simulink model "World_jessica_cs"  (R2019a)
settings: Solver=ode5  StartTime=0.0  StopTime=inf  FixedStep=1/60  RelTol=1e-3
PreLoadFcn:
  | mbxruntime.callbacks.PreLoadFcn(bdroot);
PostLoadFcn:
  | mbxruntime.callbacks.PostLoadFcn(bdroot);
InitFcn:
  | mbxruntime.callbacks.InitFcn(bdroot);
StartFcn:
  | mbxruntime.callbacks.StartFcn(bdroot);
StopFcn:
  | mbxruntime.callbacks.StopFcn(bdroot);
model workspace: external: MAT-File .\World_jessica_cs_hws.mat (data not in the file)
undefined symbols (not defined in the file or in its folder): DiscIntNeverNeededParam, InitImageOutputDir, mbxruntime, tabledata, World_jessica_cs_4acb408e0ac9f240, World_jessica_cs_800e508dbc53d9df, World_jessica_cs_Audi_A8_Sedan_1_Path_pathUniqueID, World_jessica_cs_bd1f9e0b3a3a0faa, World_jessica_cs_BMW_X5_SUV_1_Path_pathUniqueID, World_jessica_cs_BMW_X5_SUV_1_SpeedProfile_speedProfileUniqueID, World_jessica_cs_Boy_150_1_Path_pathUniqueID, World_jessica_cs_Boy_150_1_SpeedProfile_speedProfileUniqueID, World_jessica_cs_Citroen_C3_Hatchback_1_Path_pathUniqueID, World_jessica_cs_Male_CyclingCyclist_1_Path_pathUniqueID
libraries: adeye_lib x26, simulink_extras x24, simulink x2, PreScanUsefulBlocks x1
(part 5 of 7)

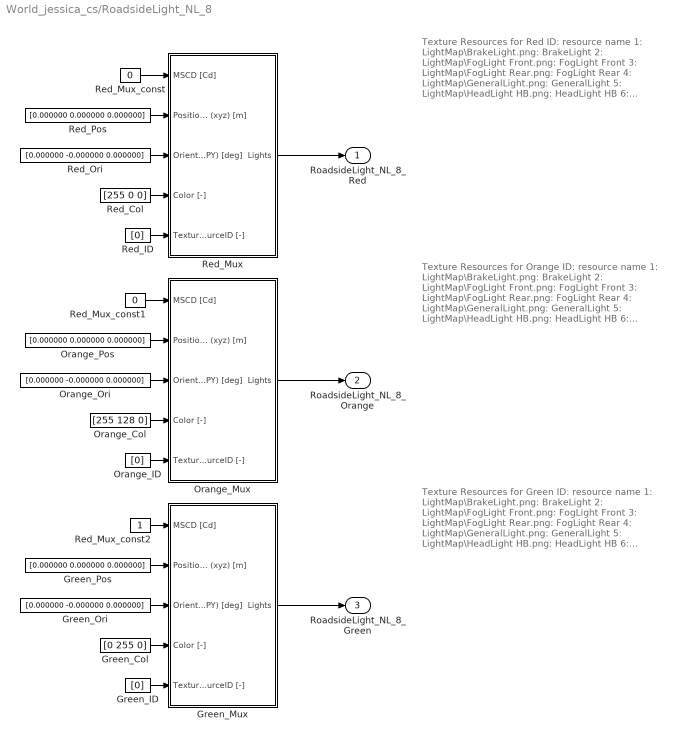
== system World_jessica_cs/RoadsideLight_NL_8 ==
  note: Texture Resources for Red
      |
      | ID: resource name
      | 1: LightMap\BrakeLight.png: BrakeLight
      | 2: LightMap\FogLight Front.png: FogLight Front
      | 3: LightMap\FogLight Rear.png: FogLight Rear
      | 4: LightMap\GeneralLight.png: GeneralLight
      | 5: LightMap\HeadLight HB.png: HeadLight HB
      | 6: LightMap\HeadLight LB.png: HeadLight LB
      | 7: LightMap\RearLight.png: RearLight
      | 8: LightMap\ReversingLight.png: ReversingLight
  note: Texture Resources for Orange
      |
      | ID: resource name
      | 1: LightMap\BrakeLight.png: BrakeLight
      | 2: LightMap\FogLight Front.png: FogLight Front
      | 3: LightMap\FogLight Rear.png: FogLight Rear
      | 4: LightMap\GeneralLight.png: GeneralLight
      | 5: LightMap\HeadLight HB.png: HeadLight HB
      | 6: LightMap\HeadLight LB.png: HeadLight LB
      | 7: LightMap\RearLight.png: RearLight
      | 8: LightMap\ReversingLight.png: ReversingLight
  note: Texture Resources for Green
      |
      | ID: resource name
      | 1: LightMap\BrakeLight.png: BrakeLight
      | 2: LightMap\FogLight Front.png: FogLight Front
      | 3: LightMap\FogLight Rear.png: FogLight Rear
      | 4: LightMap\GeneralLight.png: GeneralLight
      | 5: LightMap\HeadLight HB.png: HeadLight HB
      | 6: LightMap\HeadLight LB.png: HeadLight LB
      | 7: LightMap\RearLight.png: RearLight
      | 8: LightMap\ReversingLight.png: ReversingLight
  Green_Col : Constant  Tag=VisuLightConst  Value=[0 255 0]
  Green_ID : Constant  Tag=VisuLightConst  Value=[0]
  Green_Mux : Subsystem  Tag=mux/ActiveLight  mask(PreScan User Interface: VisuActiveLight){}
      mask help:
      | The VisuActiveLight block provides a way for detailed animation of Light Sources, such as the indicator, brake, fog and main lights of a vehicle, or a light post.
      |
      | For more information, please click Help.
      settings: DeleteFcn=PreScanBlockDeleteFcn;
      mask Help: eval('openHelp(209)')
  Green_Ori : Constant  Tag=VisuLightConst  Value=[0.000000 -0.000000 0.000000]
  Green_Pos : Constant  Tag=VisuLightConst  Value=[0.000000 0.000000 0.000000]
  Orange_Col : Constant  Tag=VisuLightConst  Value=[255 128 0]
  Orange_ID : Constant  Tag=VisuLightConst  Value=[0]
  Orange_Mux : Subsystem  Tag=mux/ActiveLight  mask(PreScan User Interface: VisuActiveLight){}
      mask help:
      | The VisuActiveLight block provides a way for detailed animation of Light Sources, such as the indicator, brake, fog and main lights of a vehicle, or a light post.
      |
      | For more information, please click Help.
      settings: DeleteFcn=PreScanBlockDeleteFcn;
      mask Help: eval('openHelp(209)')
  Orange_Ori : Constant  Tag=VisuLightConst  Value=[0.000000 -0.000000 0.000000]
  Orange_Pos : Constant  Tag=VisuLightConst  Value=[0.000000 0.000000 0.000000]
  Red_Col : Constant  Tag=VisuLightConst  Value=[255 0 0]
  Red_ID : Constant  Tag=VisuLightConst  Value=[0]
  Red_Mux : Subsystem  Tag=mux/ActiveLight  mask(PreScan User Interface: VisuActiveLight){}
      mask help:
      | The VisuActiveLight block provides a way for detailed animation of Light Sources, such as the indicator, brake, fog and main lights of a vehicle, or a light post.
      |
      | For more information, please click Help.
      settings: DeleteFcn=PreScanBlockDeleteFcn;
      mask Help: eval('openHelp(209)')
  Red_Mux_const : Constant  Tag=VisuLightConst  Value=0
  Red_Mux_const1 : Constant  Tag=VisuLightConst  Value=0
  Red_Mux_const2 : Constant  Tag=VisuLightConst
  Red_Ori : Constant  Tag=VisuLightConst  Value=[0.000000 -0.000000 0.000000]
  Red_Pos : Constant  Tag=VisuLightConst  Value=[0.000000 0.000000 0.000000]
  RoadsideLight_NL_8_Red : Outport  Tag=outport/Red  OutDataTypeStr=Bus: PRESCAN_VISULIGHTACTUATOR_DATA  SampleTime=1/60
  RoadsideLight_NL_8_Orange : Outport  Tag=outport/Orange  Port=2  OutDataTypeStr=Bus: PRESCAN_VISULIGHTACTUATOR_DATA  SampleTime=1/60
  RoadsideLight_NL_8_Green : Outport  Tag=outport/Green  Port=3  OutDataTypeStr=Bus: PRESCAN_VISULIGHTACTUATOR_DATA  SampleTime=1/60
  wires:
  Red_Mux_const/1 -> Red_Mux/1(MSCD [Cd])
  Red_Mux_const1/1 -> Orange_Mux/1(MSCD [Cd])
  Red_Mux_const2/1 -> Green_Mux/1(MSCD [Cd])
  Red_Mux/1(Lights) -> RoadsideLight_NL_8_Red/1
  Red_Pos/1 -> Red_Mux/2(Position (xyz) [m])
  Red_Ori/1 -> Red_Mux/3(Orientation (RPY) [deg])
  Red_Col/1 -> Red_Mux/4(Color [-])
  Red_ID/1 -> Red_Mux/5(TextureResourceID [-])
  Orange_Mux/1(Lights) -> RoadsideLight_NL_8_Orange/1
  Orange_Pos/1 -> Orange_Mux/2(Position (xyz) [m])
  Orange_Ori/1 -> Orange_Mux/3(Orientation (RPY) [deg])
  Orange_Col/1 -> Orange_Mux/4(Color [-])
  Orange_ID/1 -> Orange_Mux/5(TextureResourceID [-])
  Green_Mux/1(Lights) -> RoadsideLight_NL_8_Green/1
  Green_Pos/1 -> Green_Mux/2(Position (xyz) [m])
  Green_Ori/1 -> Green_Mux/3(Orientation (RPY) [deg])
  Green_Col/1 -> Green_Mux/4(Color [-])
  Green_ID/1 -> Green_Mux/5(TextureResourceID [-])

== system World_jessica_cs/RoadsideLight_NL_8_Green ==
  RoadsideLight_NL_8_Green : Inport  Tag=inport/Green  OutDataTypeStr=Bus: PRESCAN_VISULIGHTACTUATOR_DATA  SampleTime=1/60  BusOutputAsStruct=on
  Actuator : S-Function  FunctionName=sfun_VisuLightActuator  Parameters=mbxruntime.parameters.convert(UniqueID), mbxruntime.parameters.convert(LightName), mbxruntime.parameters.convert(PivotName), mbxruntime.parameters.convert(TextureResources), mbxruntime.parameters.convert(ColorsObjectName), mbxruntime.parameters.convert(MeshOnColor), mbxruntime.parameters.convert(MeshOffColor),tabledata, TimeStep  SFunctionDeploymentMode=off  EnableBusSupport=off  mask(PreScan Sink Block: VisuActiveLight){UniqueID=4882, LightName=RoadsideLight_NL_8.LightActuator_2_Green_ActiveLight, PivotName=RoadsideLight_NL_8.Green, TextureResources={ '1' 'LightMap\BrakeLight.png' '2' 'LightMap\FogLight Front.png' '3' 'LightMap\FogLight Rear.png' '4' 'LightMap\GeneralLight.png' '5' 'LightMap\HeadLight HB.png' '6' 'LightMap\HeadLight LB.png' '7' 'LightMap\RearLight.png' '8' 'LightMap\ReversingLight.png'}, ColorsObjectName=RoadsideLight_NL_8.Green, MeshOnColor=[0  100    0  255    0  100    0  255  102  102  102  255    0  510    0  255], MeshOffColor=[0  100    0  255    0  100    0  255  102  102  102  255    0    0    0  255], TimeStep=1/60}
      mask prompts: UniqueID "Parent Unique Identifier"; LightName "Light"; PivotName "Pivot"; TextureResources "Texture Resources"; ColorsObjectName "Light Fixture Color Object"; MeshOnColor "Light Fixture On Color"; MeshOffColor "Light Fixture Off Color"; TimeStep "Simulink time step"
      mask help:
      | The VisuActiveLight block provides a way for detailed animation of Light Sources, such as the indicator, brake, fog and main lights of a vehicle, or a light post.
      |
      | For more information, please click Help.
      mask init:
      | [tabledata] = mbxruntime.parameters.table(UniqueID,LightName,PivotName,TextureResources,ColorsObjectName,MeshOnColor,MeshOffColor);
      mask Help: eval('openHelp(209)')
      mask Display: image(imread('HeadLight.png'))
  wires:
  RoadsideLight_NL_8_Green/1 -> Actuator/1

== system World_jessica_cs/RoadsideLight_NL_8_Orange ==
  RoadsideLight_NL_8_Orange : Inport  Tag=inport/Orange  OutDataTypeStr=Bus: PRESCAN_VISULIGHTACTUATOR_DATA  SampleTime=1/60  BusOutputAsStruct=on
  Actuator : S-Function  FunctionName=sfun_VisuLightActuator  Parameters=mbxruntime.parameters.convert(UniqueID), mbxruntime.parameters.convert(LightName), mbxruntime.parameters.convert(PivotName), mbxruntime.parameters.convert(TextureResources), mbxruntime.parameters.convert(ColorsObjectName), mbxruntime.parameters.convert(MeshOnColor), mbxruntime.parameters.convert(MeshOffColor),tabledata, TimeStep  SFunctionDeploymentMode=off  EnableBusSupport=off  mask(PreScan Sink Block: VisuActiveLight){UniqueID=4882, LightName=RoadsideLight_NL_8.LightActuator_1_Orange_ActiveLight, PivotName=RoadsideLight_NL_8.Orange, TextureResources={ '1' 'LightMap\BrakeLight.png' '2' 'LightMap\FogLight Front.png' '3' 'LightMap\FogLight Rear.png' '4' 'LightMap\GeneralLight.png' '5' 'LightMap\HeadLight HB.png' '6' 'LightMap\HeadLight LB.png' '7' 'LightMap\RearLight.png' '8' 'LightMap\ReversingLight.png'}, ColorsObjectName=RoadsideLight_NL_8.Orange, MeshOnColor=[100   50    0  255  100   50    0  255  102  102  102  255  510  256    0  255], MeshOffColor=[100   50    0  255  100   50    0  255  102  102  102  255    0    0    0  255], TimeStep=1/60}
      mask prompts: UniqueID "Parent Unique Identifier"; LightName "Light"; PivotName "Pivot"; TextureResources "Texture Resources"; ColorsObjectName "Light Fixture Color Object"; MeshOnColor "Light Fixture On Color"; MeshOffColor "Light Fixture Off Color"; TimeStep "Simulink time step"
      mask help:
      | The VisuActiveLight block provides a way for detailed animation of Light Sources, such as the indicator, brake, fog and main lights of a vehicle, or a light post.
      |
      | For more information, please click Help.
      mask init:
      | [tabledata] = mbxruntime.parameters.table(UniqueID,LightName,PivotName,TextureResources,ColorsObjectName,MeshOnColor,MeshOffColor);
      mask Help: eval('openHelp(209)')
      mask Display: image(imread('HeadLight.png'))
  wires:
  RoadsideLight_NL_8_Orange/1 -> Actuator/1

== system World_jessica_cs/RoadsideLight_NL_8_Red ==
  RoadsideLight_NL_8_Red : Inport  Tag=inport/Red  OutDataTypeStr=Bus: PRESCAN_VISULIGHTACTUATOR_DATA  SampleTime=1/60  BusOutputAsStruct=on
  Actuator : S-Function  FunctionName=sfun_VisuLightActuator  Parameters=mbxruntime.parameters.convert(UniqueID), mbxruntime.parameters.convert(LightName), mbxruntime.parameters.convert(PivotName), mbxruntime.parameters.convert(TextureResources), mbxruntime.parameters.convert(ColorsObjectName), mbxruntime.parameters.convert(MeshOnColor), mbxruntime.parameters.convert(MeshOffColor),tabledata, TimeStep  SFunctionDeploymentMode=off  EnableBusSupport=off  mask(PreScan Sink Block: VisuActiveLight){UniqueID=4882, LightName=RoadsideLight_NL_8.LightActuator_0_Red_ActiveLight, PivotName=RoadsideLight_NL_8.Red, TextureResources={ '1' 'LightMap\BrakeLight.png' '2' 'LightMap\FogLight Front.png' '3' 'LightMap\FogLight Rear.png' '4' 'LightMap\GeneralLight.png' '5' 'LightMap\HeadLight HB.png' '6' 'LightMap\HeadLight LB.png' '7' 'LightMap\RearLight.png' '8' 'LightMap\ReversingLight.png'}, ColorsObjectName=RoadsideLight_NL_8.Red, MeshOnColor=[100    0    0  255  100    0    0  255  102  102  102  255  510    0    0  255], MeshOffColor=[100    0    0  255  100    0    0  255  102  102  102  255    0    0    0  255], TimeStep=1/60}
      mask prompts: UniqueID "Parent Unique Identifier"; LightName "Light"; PivotName "Pivot"; TextureResources "Texture Resources"; ColorsObjectName "Light Fixture Color Object"; MeshOnColor "Light Fixture On Color"; MeshOffColor "Light Fixture Off Color"; TimeStep "Simulink time step"
      mask help:
      | The VisuActiveLight block provides a way for detailed animation of Light Sources, such as the indicator, brake, fog and main lights of a vehicle, or a light post.
      |
      | For more information, please click Help.
      mask init:
      | [tabledata] = mbxruntime.parameters.table(UniqueID,LightName,PivotName,TextureResources,ColorsObjectName,MeshOnColor,MeshOffColor);
      mask Help: eval('openHelp(209)')
      mask Display: image(imread('HeadLight.png'))
  wires:
  RoadsideLight_NL_8_Red/1 -> Actuator/1

== system World_jessica_cs/SELF_Audi_A8_Sedan_1 ==
  Sensor : S-Function  FunctionName=sfun_SelfSensor  Parameters=UniqueID, TimeStep  SFunctionDeploymentMode=off  EnableBusSupport=off  mask(PreScan Source Block: SELF){UniqueID=4533, TimeStep=1/60}
      mask prompts: UniqueID "Auto-Assigned: Unique ID"; TimeStep "Auto-Assigned: Upload Period [s]"
      mask help:
      | The SELF port shows (state) information of the actor itself. The outputs are position in the experiment's axis system and the GPS coordinates, and the object's absolute velocity and compass heading.
      |
      | For more information, please click Help.
      mask Help: eval('openHelp(462)')
      mask Display: image(imread('GPS.png'))
  SELF_Audi_A8_Sedan_1 : Outport  Tag=outport/SelfPort  OutDataTypeStr=Bus: PRESCAN_SELFSENSORDATA  PortDimensions=1  SampleTime=1/60
  wires:
  Sensor/1 -> SELF_Audi_A8_Sedan_1/1

== system World_jessica_cs/SELF_BMW_X5_SUV_1 ==
  Sensor : S-Function  FunctionName=sfun_SelfSensor  Parameters=UniqueID, TimeStep  SFunctionDeploymentMode=off  EnableBusSupport=off  mask(PreScan Source Block: SELF){UniqueID=5671, TimeStep=1/60}
      mask prompts: UniqueID "Auto-Assigned: Unique ID"; TimeStep "Auto-Assigned: Upload Period [s]"
      mask help:
      | The SELF port shows (state) information of the actor itself. The outputs are position in the experiment's axis system and the GPS coordinates, and the object's absolute velocity and compass heading.
      |
      | For more information, please click Help.
      mask Help: eval('openHelp(462)')
      mask Display: image(imread('GPS.png'))
  SELF_BMW_X5_SUV_1 : Outport  Tag=outport/SelfPort  OutDataTypeStr=Bus: PRESCAN_SELFSENSORDATA  PortDimensions=1  SampleTime=1/60
  wires:
  Sensor/1 -> SELF_BMW_X5_SUV_1/1

== system World_jessica_cs/SELF_Boy_150_1 ==
  Sensor : S-Function  FunctionName=sfun_SelfSensor  Parameters=UniqueID, TimeStep  SFunctionDeploymentMode=off  EnableBusSupport=off  mask(PreScan Source Block: SELF){UniqueID=4541, TimeStep=1/60}
      mask prompts: UniqueID "Auto-Assigned: Unique ID"; TimeStep "Auto-Assigned: Upload Period [s]"
      mask help:
      | The SELF port shows (state) information of the actor itself. The outputs are position in the experiment's axis system and the GPS coordinates, and the object's absolute velocity and compass heading.
      |
      | For more information, please click Help.
      mask Help: eval('openHelp(462)')
      mask Display: image(imread('GPS.png'))
  SELF_Boy_150_1 : Outport  Tag=outport/SelfPort  OutDataTypeStr=Bus: PRESCAN_SELFSENSORDATA  PortDimensions=1  SampleTime=1/60
  wires:
  Sensor/1 -> SELF_Boy_150_1/1

== system World_jessica_cs/SELF_Citroen_C3_Hatchback_1 ==
  Sensor : S-Function  FunctionName=sfun_SelfSensor  Parameters=UniqueID, TimeStep  SFunctionDeploymentMode=off  EnableBusSupport=off  mask(PreScan Source Block: SELF){UniqueID=4537, TimeStep=1/60}
      mask prompts: UniqueID "Auto-Assigned: Unique ID"; TimeStep "Auto-Assigned: Upload Period [s]"
      mask help:
      | The SELF port shows (state) information of the actor itself. The outputs are position in the experiment's axis system and the GPS coordinates, and the object's absolute velocity and compass heading.
      |
      | For more information, please click Help.
      mask Help: eval('openHelp(462)')
      mask Display: image(imread('GPS.png'))
  SELF_Citroen_C3_Hatchback_1 : Outport  Tag=outport/SelfPort  OutDataTypeStr=Bus: PRESCAN_SELFSENSORDATA  PortDimensions=1  SampleTime=1/60
  wires:
  Sensor/1 -> SELF_Citroen_C3_Hatchback_1/1

== system World_jessica_cs/SELF_Male_CyclingCyclist_1 ==
  Sensor : S-Function  FunctionName=sfun_SelfSensor  Parameters=UniqueID, TimeStep  SFunctionDeploymentMode=off  EnableBusSupport=off  mask(PreScan Source Block: SELF){UniqueID=4545, TimeStep=1/60}
      mask prompts: UniqueID "Auto-Assigned: Unique ID"; TimeStep "Auto-Assigned: Upload Period [s]"
      mask help:
      | The SELF port shows (state) information of the actor itself. The outputs are position in the experiment's axis system and the GPS coordinates, and the object's absolute velocity and compass heading.
      |
      | For more information, please click Help.
      mask Help: eval('openHelp(462)')
      mask Display: image(imread('GPS.png'))
  SELF_Male_CyclingCyclist_1 : Outport  Tag=outport/SelfPort  OutDataTypeStr=Bus: PRESCAN_SELFSENSORDATA  PortDimensions=1  SampleTime=1/60
  wires:
  Sensor/1 -> SELF_Male_CyclingCyclist_1/1

== system World_jessica_cs/STATE_Audi_A8_Sedan_1_bus ==
  STATE_Audi_A8_Sedan_1_bus : Inport  Tag=inport/StatePort  OutDataTypeStr=Bus: PRESCAN_STATEACTUATORDATA  PortDimensions=1  SampleTime=1/60  BusOutputAsStruct=on
  Actuator : S-Function  FunctionName=sfun_StateActuator  Parameters=UniqueID, TimeStep  SFunctionDeploymentMode=off  EnableBusSupport=off  mask(PreScan Sink Block: State){UniqueID=4533, TimeStep=1/60}
      mask prompts: UniqueID "Auto-Assigned: Unique ID"; TimeStep "Auto-Assigned: Upload Period [s]"
      mask help:
      | The Actor State contains a vector signal of size (9x1), containing the following signals:
      |
      | -  Position    	(x,y,z)             	[m]
      | -  Velocity    	(vx,vy,vz)         	[m/s]
      | -  Angles       	(Roll, Pitch, Yaw)	[rad]
      |
      | The Actor state is defined in the global axis system.
      | The state is superponed on the Initial position defined in the GUI.
      |
      | For more information, please click Help.
      mask Help: eval('openHelp(222)')
      mask Display: image(imread('State.png'))
  wires:
  STATE_Audi_A8_Sedan_1_bus/1 -> Actuator/1

== system World_jessica_cs/STATE_BMW_X5_SUV_1_bus ==
  STATE_BMW_X5_SUV_1_bus : Inport  Tag=inport/StatePort  OutDataTypeStr=Bus: PRESCAN_STATEACTUATORDATA  PortDimensions=1  SampleTime=1/60  BusOutputAsStruct=on
  Actuator : S-Function  FunctionName=sfun_StateActuator  Parameters=UniqueID, TimeStep  SFunctionDeploymentMode=off  EnableBusSupport=off  mask(PreScan Sink Block: State){UniqueID=5671, TimeStep=1/60}
      mask prompts: UniqueID "Auto-Assigned: Unique ID"; TimeStep "Auto-Assigned: Upload Period [s]"
      mask help:
      | The Actor State contains a vector signal of size (9x1), containing the following signals:
      |
      | -  Position    	(x,y,z)             	[m]
      | -  Velocity    	(vx,vy,vz)         	[m/s]
      | -  Angles       	(Roll, Pitch, Yaw)	[rad]
      |
      | The Actor state is defined in the global axis system.
      | The state is superponed on the Initial position defined in the GUI.
      |
      | For more information, please click Help.
      mask Help: eval('openHelp(222)')
      mask Display: image(imread('State.png'))
  wires:
  STATE_BMW_X5_SUV_1_bus/1 -> Actuator/1

== system World_jessica_cs/STATE_Boy_150_1_bus ==
  STATE_Boy_150_1_bus : Inport  Tag=inport/StatePort  OutDataTypeStr=Bus: PRESCAN_STATEACTUATORDATA  PortDimensions=1  SampleTime=1/60  BusOutputAsStruct=on
  Actuator : S-Function  FunctionName=sfun_StateActuator  Parameters=UniqueID, TimeStep  SFunctionDeploymentMode=off  EnableBusSupport=off  mask(PreScan Sink Block: State){UniqueID=4541, TimeStep=1/60}
      mask prompts: UniqueID "Auto-Assigned: Unique ID"; TimeStep "Auto-Assigned: Upload Period [s]"
      mask help:
      | The Actor State contains a vector signal of size (9x1), containing the following signals:
      |
      | -  Position    	(x,y,z)             	[m]
      | -  Velocity    	(vx,vy,vz)         	[m/s]
      | -  Angles       	(Roll, Pitch, Yaw)	[rad]
      |
      | The Actor state is defined in the global axis system.
      | The state is superponed on the Initial position defined in the GUI.
      |
      | For more information, please click Help.
      mask Help: eval('openHelp(222)')
      mask Display: image(imread('State.png'))
  wires:
  STATE_Boy_150_1_bus/1 -> Actuator/1

== system World_jessica_cs/STATE_Citroen_C3_Hatchback_1_bus ==
  STATE_Citroen_C3_Hatchback_1_bus : Inport  Tag=inport/StatePort  OutDataTypeStr=Bus: PRESCAN_STATEACTUATORDATA  PortDimensions=1  SampleTime=1/60  BusOutputAsStruct=on
  Actuator : S-Function  FunctionName=sfun_StateActuator  Parameters=UniqueID, TimeStep  SFunctionDeploymentMode=off  EnableBusSupport=off  mask(PreScan Sink Block: State){UniqueID=4537, TimeStep=1/60}
      mask prompts: UniqueID "Auto-Assigned: Unique ID"; TimeStep "Auto-Assigned: Upload Period [s]"
      mask help:
      | The Actor State contains a vector signal of size (9x1), containing the following signals:
      |
      | -  Position    	(x,y,z)             	[m]
      | -  Velocity    	(vx,vy,vz)         	[m/s]
      | -  Angles       	(Roll, Pitch, Yaw)	[rad]
      |
      | The Actor state is defined in the global axis system.
      | The state is superponed on the Initial position defined in the GUI.
      |
      | For more information, please click Help.
      mask Help: eval('openHelp(222)')
      mask Display: image(imread('State.png'))
  wires:
  STATE_Citroen_C3_Hatchback_1_bus/1 -> Actuator/1

== system World_jessica_cs/STATE_Male_CyclingCyclist_1_bus ==
  STATE_Male_CyclingCyclist_1_bus : Inport  Tag=inport/StatePort  OutDataTypeStr=Bus: PRESCAN_STATEACTUATORDATA  PortDimensions=1  SampleTime=1/60  BusOutputAsStruct=on
  Actuator : S-Function  FunctionName=sfun_StateActuator  Parameters=UniqueID, TimeStep  SFunctionDeploymentMode=off  EnableBusSupport=off  mask(PreScan Sink Block: State){UniqueID=4545, TimeStep=1/60}
      mask prompts: UniqueID "Auto-Assigned: Unique ID"; TimeStep "Auto-Assigned: Upload Period [s]"
      mask help:
      | The Actor State contains a vector signal of size (9x1), containing the following signals:
      |
      | -  Position    	(x,y,z)             	[m]
      | -  Velocity    	(vx,vy,vz)         	[m/s]
      | -  Angles       	(Roll, Pitch, Yaw)	[rad]
      |
      | The Actor state is defined in the global axis system.
      | The state is superponed on the Initial position defined in the GUI.
      |
      | For more information, please click Help.
      mask Help: eval('openHelp(222)')
      mask Display: image(imread('State.png'))
  wires:
  STATE_Male_CyclingCyclist_1_bus/1 -> Actuator/1

== system World_jessica_cs/ScenarioEngine ==
  Clock : Clock
  sfun_ScenarioEngine : S-Function  FunctionName=sfun_ScenarioEngine  Parameters=TimeStep  SFunctionDeploymentMode=off  EnableBusSupport=off
  wires:
  Clock/1 -> sfun_ScenarioEngine/1

== system World_jessica_cs/Synchronizer ==
  Bus Selector1 : BusSelector  OutputSignals=FederateStopped
  Stop Simulation : Stop
  sfun_Synchronizer : S-Function  FunctionName=sfun_Synchronizer  Parameters=SampleTime  SFunctionDeploymentMode=off  EnableBusSupport=off  mask(Legacy Function){SFunctionSpec=void prescan_synchronizer_outputFcn(void ** work1, PRESCAN_SYNCHRONIZEDATA y1[1]), SampleTime=TimeStep, ShowSpec=on}
      mask prompts: SampleTime "Sample time (-1 for inherited):"; ShowSpec "Display function specification"
      mask help:
      | This block allows you to call the legacy functions specified by the following Legacy Code Tool definition:
      | def.SFunctionName = 'sfun_Synchronizer';
      | def.OutputFcnSpec = 'void prescan_synchronizer_outputFcn(void ** work1, PRESCAN_SYNCHRONIZEDATA y1[1])';
      | def.StartFcnSpec = 'void prescan_synchronizer_startFcn(void ** work1)';
      | def.TerminateFcnSpec = 'void prescan_synchronizer_terminateFcn(void ** work1)';
      | def.HeaderFiles = {'prescan_synchronizer_data.h'};
      | def.HostLibFiles = {'sensorinterfaced.lib'};
      | def.IncPaths = {'src', 'C:\prescandev\vislibrary\vis\..\pimp\include\sensors\InterfaceRTW'};
      | def.SrcPaths = {'src'};
      | def.LibPaths = {'C:\\prescandev\\vislibrary_build\lib'};
      | def.SampleTime = 'parameterized';
      | def.Options.language = 'C';
      mask Help: <p>This block was generated automatically by the Legacy Code Tool. For detailed help on this tool, call<a href="matlab:legacy_code('help')"> legacy_code('help')</a>.</p>
      mask Callback ShowSpec:
      | if strcmp(get_param(gcbh, 'ShowSpec'), 'on')
      |   set_param(gcbh, 'MaskDisplay', sprintf('fprintf(''%s'');', get_param(gcbh, 'SFunctionSpec')));
      | else
      |   set_param(gcbh, 'MaskDisplay', sprintf('fprintf(''%s'');', get_param(gcbh, 'FunctionName')));
      | end
      mask Display: fprintf('void prescan_synchronizer_outputFcn(void ** work1, PRESCAN_SYNCHRONIZEDATA y1[1])');
  wires:
  Bus Selector1/1 -> Stop Simulation/1  "<FederateStopped>"
  sfun_Synchronizer/1 -> Bus Selector1/1

== system World_jessica_cs/VISUColorRegion_Lower_Body_Boy_150_1 ==
  VISUColorRegion_Lower_Body_Boy_150_1 : Inport  Tag=inport/ColorRegion  OutDataTypeStr=Bus: PRESCAN_COLOR_DATA  PortDimensions=1  SampleTime=1/60  BusOutputAsStruct=on
  Actuator : S-Function  FunctionName=sfun_ColorActuator  Parameters=mbxruntime.parameters.convert(UniqueID), mbxruntime.parameters.convert(WorldModelSubPath),tabledata, TimeStep  SFunctionDeploymentMode=off  EnableBusSupport=off  mask(PreScan Sink Block: VisuTextureColor){UniqueID=4541, WorldModelSubPath=/recolorRegion:name=Lower Body/targetColor, TimeStep=1/60}
      mask prompts: UniqueID "Parent Unique Identifier (auto-generated)"; WorldModelSubPath "WM SubPath(auto-generated)"; TimeStep "Simulink time step"
      mask help:
      | The VisuTextureColor block provides a way to adapt the color of a vehicle.
      |
      | For more information, please click Help.
      mask init:
      | [tabledata] = mbxruntime.parameters.table(UniqueID,WorldModelSubPath);
      mask Help: eval('openHelp(230)')
      mask Display: image(imread('TextureColor.png'))
  wires:
  VISUColorRegion_Lower_Body_Boy_150_1/1 -> Actuator/1

== system World_jessica_cs/VISUColorRegion_Shoes_Boy_150_1 ==
  VISUColorRegion_Shoes_Boy_150_1 : Inport  Tag=inport/ColorRegion  OutDataTypeStr=Bus: PRESCAN_COLOR_DATA  PortDimensions=1  SampleTime=1/60  BusOutputAsStruct=on
  Actuator : S-Function  FunctionName=sfun_ColorActuator  Parameters=mbxruntime.parameters.convert(UniqueID), mbxruntime.parameters.convert(WorldModelSubPath),tabledata, TimeStep  SFunctionDeploymentMode=off  EnableBusSupport=off  mask(PreScan Sink Block: VisuTextureColor){UniqueID=4541, WorldModelSubPath=/recolorRegion:name=Shoes/targetColor, TimeStep=1/60}
      mask prompts: UniqueID "Parent Unique Identifier (auto-generated)"; WorldModelSubPath "WM SubPath(auto-generated)"; TimeStep "Simulink time step"
      mask help:
      | The VisuTextureColor block provides a way to adapt the color of a vehicle.
      |
      | For more information, please click Help.
      mask init:
      | [tabledata] = mbxruntime.parameters.table(UniqueID,WorldModelSubPath);
      mask Help: eval('openHelp(230)')
      mask Display: image(imread('TextureColor.png'))
  wires:
  VISUColorRegion_Shoes_Boy_150_1/1 -> Actuator/1

== system World_jessica_cs/VISUColorRegion_Upper_Body_Boy_150_1 ==
  VISUColorRegion_Upper_Body_Boy_150_1 : Inport  Tag=inport/ColorRegion  OutDataTypeStr=Bus: PRESCAN_COLOR_DATA  PortDimensions=1  SampleTime=1/60  BusOutputAsStruct=on
  Actuator : S-Function  FunctionName=sfun_ColorActuator  Parameters=mbxruntime.parameters.convert(UniqueID), mbxruntime.parameters.convert(WorldModelSubPath),tabledata, TimeStep  SFunctionDeploymentMode=off  EnableBusSupport=off  mask(PreScan Sink Block: VisuTextureColor){UniqueID=4541, WorldModelSubPath=/recolorRegion:name=Upper Body/targetColor, TimeStep=1/60}
      mask prompts: UniqueID "Parent Unique Identifier (auto-generated)"; WorldModelSubPath "WM SubPath(auto-generated)"; TimeStep "Simulink time step"
      mask help:
      | The VisuTextureColor block provides a way to adapt the color of a vehicle.
      |
      | For more information, please click Help.
      mask init:
      | [tabledata] = mbxruntime.parameters.table(UniqueID,WorldModelSubPath);
      mask Help: eval('openHelp(230)')
      mask Display: image(imread('TextureColor.png'))
  wires:
  VISUColorRegion_Upper_Body_Boy_150_1/1 -> Actuator/1

== system World_jessica_cs/Audi_A8_Sedan_1/SELF_Demux ==
  SELF : Inport  OutDataTypeStr=Bus: PRESCAN_SELFSENSORDATA
  Bus Selector : BusSelector  OutputSignals=PositionX,PositionY,PositionZ,OrientationRoll,OrientationPitch,OrientationYaw,Velocity,Yaw_rate,Lat,Long,Alt
  Demux2 : Demux  Outputs=3
  Gain : Gain  Gain=180/pi
  Gain1 : Gain  Gain=180/pi
  Vector Concatenate1 : Concatenate  NumInputs=3
  compas converter : Subsystem
  x [m] : Outport
  y [m] : Outport  Port=2
  z [m] : Outport  Port=3
  rotx [deg] : Outport  Port=4
  roty [deg] : Outport  Port=5
  rotz [deg] : Outport  Port=6
  GPS lat [deg] : Outport  Port=7
  GPS long [deg] : Outport  Port=8
  GPS alt [m] : Outport  Port=9
  velocity [m/s] : Outport  Port=10
  heading [deg] : Outport  Port=11
  yaw rate [deg/s] : Outport  Port=12
  wires:
  Bus Selector/11 -> GPS alt [m]/1  "<Alt>"
  Bus Selector/10 -> GPS long [deg]/1  "<Long>"
  Bus Selector/9 -> GPS lat [deg]/1  "<Lat>"
  Bus Selector/8 -> Gain1/1  "<Yaw_rate>"
  Bus Selector/7 -> velocity [m/s]/1  "<Velocity>"
  Bus Selector/6 -> compas converter/1(rotz [rad]), Vector Concatenate1/3  "<OrientationYaw>"
  Bus Selector/5 -> Vector Concatenate1/2  "<OrientationPitch>"
  Bus Selector/4 -> Vector Concatenate1/1  "<OrientationRoll>"
  Vector Concatenate1/1 -> Gain/1
  Bus Selector/3 -> z [m]/1  "<PositionZ>"
  Bus Selector/2 -> y [m]/1  "<PositionY>"
  Bus Selector/1 -> x [m]/1  "<PositionX>"
  SELF/1 -> Bus Selector/1
  Gain/1 -> Demux2/1
  Demux2/1 -> rotx [deg]/1
  Demux2/2 -> roty [deg]/1
  Demux2/3 -> rotz [deg]/1
  compas converter/1(heading [deg]) -> heading [deg]/1
  Gain1/1 -> yaw rate [deg/s]/1

== system World_jessica_cs/BMW_X5_SUV_1/Camera_1_CM_Demux ==
  In1 : Inport
  Selector : Selector  NumberOfDimensions=2  InputPortWidth=3  IndexOptions=Index vector (dialog),Index vector (dialog)  Indices=-1,1:hres  OutputSizes=1,1
  Selector1 : Selector  NumberOfDimensions=2  InputPortWidth=3  IndexOptions=Index vector (dialog),Index vector (dialog)  Indices=-1,hres+1:hres*2  OutputSizes=1,1
  Selector2 : Selector  NumberOfDimensions=2  InputPortWidth=3  IndexOptions=Index vector (dialog),Index vector (dialog)  Indices=-1,hres*2+1:hres*3  OutputSizes=1,1
  R : Outport
  G : Outport  Port=2
  B : Outport  Port=3
  wires:
  In1/1 -> Selector1/1, Selector/1, Selector2/1
  Selector/1 -> R/1
  Selector1/1 -> G/1
  Selector2/1 -> B/1

== system World_jessica_cs/BMW_X5_SUV_1/Camera_2_CM_Demux ==
  In1 : Inport
  Selector : Selector  NumberOfDimensions=2  InputPortWidth=3  IndexOptions=Index vector (dialog),Index vector (dialog)  Indices=-1,1:hres  OutputSizes=1,1
  Selector1 : Selector  NumberOfDimensions=2  InputPortWidth=3  IndexOptions=Index vector (dialog),Index vector (dialog)  Indices=-1,hres+1:hres*2  OutputSizes=1,1
  Selector2 : Selector  NumberOfDimensions=2  InputPortWidth=3  IndexOptions=Index vector (dialog),Index vector (dialog)  Indices=-1,hres*2+1:hres*3  OutputSizes=1,1
  R : Outport
  G : Outport  Port=2
  B : Outport  Port=3
  wires:
  In1/1 -> Selector1/1, Selector/1, Selector2/1
  Selector/1 -> R/1
  Selector1/1 -> G/1
  Selector2/1 -> B/1

== system World_jessica_cs/BMW_X5_SUV_1/Camera_tl_CM_Demux ==
  In1 : Inport
  Selector : Selector  NumberOfDimensions=2  InputPortWidth=3  IndexOptions=Index vector (dialog),Index vector (dialog)  Indices=-1,1:hres  OutputSizes=1,1
  Selector1 : Selector  NumberOfDimensions=2  InputPortWidth=3  IndexOptions=Index vector (dialog),Index vector (dialog)  Indices=-1,hres+1:hres*2  OutputSizes=1,1
  Selector2 : Selector  NumberOfDimensions=2  InputPortWidth=3  IndexOptions=Index vector (dialog),Index vector (dialog)  Indices=-1,hres*2+1:hres*3  OutputSizes=1,1
  R : Outport
  G : Outport  Port=2
  B : Outport  Port=3
  wires:
  In1/1 -> Selector1/1, Selector/1, Selector2/1
  Selector/1 -> R/1
  Selector1/1 -> G/1
  Selector2/1 -> B/1

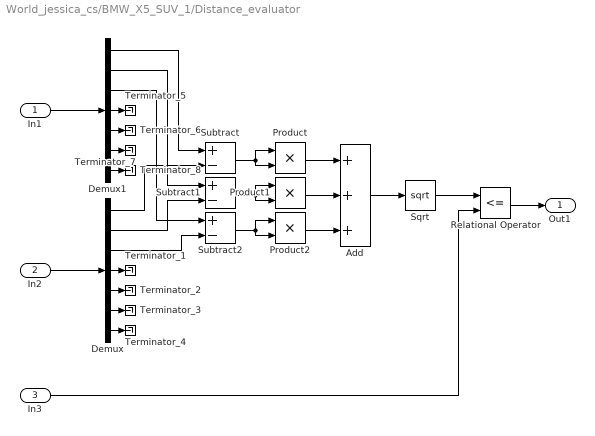
== system World_jessica_cs/BMW_X5_SUV_1/Distance_evaluator ==
  In1 : Inport
  In2 : Inport  Port=2
  In3 : Inport  Port=3
  Add : Sum  Inputs=3
  Demux : Demux  Outputs=7
  Demux1 : Demux  Outputs=7
  Product : Product
  Product1 : Product
  Product2 : Product
  Relational Operator : RelationalOperator  Operator=<=  OutDataTypeStr=boolean  RndMeth=Simplest
  Sqrt : Sqrt  SaturateOnIntegerOverflow=on
  Subtract : Sum  Inputs=+-
  Subtract1 : Sum  Inputs=+-
  Subtract2 : Sum  Inputs=+-
  Terminator_{1..8} (8 alike) : Terminator
  Out1 : Outport
  wires:
  Relational Operator/1 -> Out1/1
  In1/1 -> Demux1/1
  In2/1 -> Demux/1
  Demux1/1 -> Subtract/1
  Demux1/2 -> Subtract1/1
  Demux1/3 -> Subtract2/1
  Demux/1 -> Subtract/2
  Demux/2 -> Subtract1/2
  Demux/3 -> Subtract2/2
  Subtract/1 -> Product/1, Product/2
  Subtract1/1 -> Product1/1, Product1/2
  Subtract2/1 -> Product2/1, Product2/2
  Product/1 -> Add/1
  Product1/1 -> Add/2
  Product2/1 -> Add/3
  Add/1 -> Sqrt/1
  Sqrt/1 -> Relational Operator/1
  In3/1 -> Relational Operator/2
  Demux/4 -> Terminator_1/1
  Demux/5 -> Terminator_2/1
  Demux/6 -> Terminator_3/1
  Demux/7 -> Terminator_4/1
  Demux1/4 -> Terminator_5/1
  Demux1/5 -> Terminator_6/1
  Demux1/6 -> Terminator_7/1
  Demux1/7 -> Terminator_8/1

== system World_jessica_cs/BMW_X5_SUV_1/Fault Injection Camera1 ==
  In1 : Inport
  In2 : Inport  Port=2
  In3 : Inport  Port=3
  In4 : Inport  Port=4
  In5 : Inport  Port=5
  In6 : Inport  Port=6
  In7 : Inport  Port=7
  If : If
  If Action Subsystem : Subsystem  TreatAsAtomicUnit=on
  If Action Subsystem1 : Subsystem  TreatAsAtomicUnit=on
  Merge : Merge
  Merge1 : Merge
  Merge2 : Merge
  Out1 : Outport
  Out2 : Outport  Port=2
  Out3 : Outport  Port=3
  wires:
  If/1 -> If Action Subsystem1/Action
  If/2 -> If Action Subsystem/Action
  In7/1 -> If/1
  In1/1 -> If Action Subsystem1/1(In2)
  In2/1 -> If Action Subsystem1/2(In3)
  In3/1 -> If Action Subsystem1/3(In4)
  In4/1 -> If Action Subsystem/1(In1), If Action Subsystem1/4(In5)
  In5/1 -> If Action Subsystem/2(In2), If Action Subsystem1/5(In6)
  In6/1 -> If Action Subsystem/3(In3), If Action Subsystem1/6(In7)
  If Action Subsystem1/1(Out2) -> Merge/2
  If Action Subsystem1/2(Out3) -> Merge1/2
  If Action Subsystem1/3(Out4) -> Merge2/2
  Merge/1 -> Out1/1
  If Action Subsystem/1(Out1) -> Merge/1
  If Action Subsystem/2(Out2) -> Merge1/1
  If Action Subsystem/3(Out3) -> Merge2/1
  Merge1/1 -> Out2/1
  Merge2/1 -> Out3/1

== system World_jessica_cs/BMW_X5_SUV_1/Frequency evaluator ==
  In1 : Inport
  Add : Sum  Inputs=+-
  Clock2 : Clock
  Constant : Constant
  Divide : Product  Inputs=*/
  Memory : Memory
  Relational Operator : RelationalOperator  OutDataTypeStr=boolean  RndMeth=Simplest
  Switch : Switch  Criteria=u2 > Threshold
  Out1 : Outport
  wires:
  Memory/1 -> Switch/3, Add/2
  Switch/1 -> Memory/1
  Add/1 -> Relational Operator/1
  Relational Operator/1 -> Switch/2, Out1/1
  Clock2/1 -> Add/1, Switch/1
  In1/1 -> Divide/2
  Constant/1 -> Divide/1
  Divide/1 -> Relational Operator/2

== system World_jessica_cs/BMW_X5_SUV_1/Frequency evaluator1 ==
  In1 : Inport
  Add : Sum  Inputs=+-
  Clock2 : Clock
  Constant : Constant
  Divide : Product  Inputs=*/
  Memory : Memory
  Relational Operator : RelationalOperator  OutDataTypeStr=boolean  RndMeth=Simplest
  Switch : Switch  Criteria=u2 > Threshold
  Out1 : Outport
  wires:
  Memory/1 -> Switch/3, Add/2
  Switch/1 -> Memory/1
  Add/1 -> Relational Operator/1
  Relational Operator/1 -> Switch/2, Out1/1
  Clock2/1 -> Add/1, Switch/1
  In1/1 -> Divide/2
  Constant/1 -> Divide/1
  Divide/1 -> Relational Operator/2

== system World_jessica_cs/BMW_X5_SUV_1/Frequency evaluator2 ==
  In1 : Inport
  Add : Sum  Inputs=+-
  Clock2 : Clock
  Constant : Constant
  Divide : Product  Inputs=*/
  Memory : Memory
  Relational Operator : RelationalOperator  OutDataTypeStr=boolean  RndMeth=Simplest
  Switch : Switch  Criteria=u2 > Threshold
  Out1 : Outport
  wires:
  Memory/1 -> Switch/3, Add/2
  Switch/1 -> Memory/1
  Add/1 -> Relational Operator/1
  Relational Operator/1 -> Switch/2, Out1/1
  Clock2/1 -> Add/1, Switch/1
  In1/1 -> Divide/2
  Constant/1 -> Divide/1
  Divide/1 -> Relational Operator/2

== system World_jessica_cs/BMW_X5_SUV_1/Frequency evaluator3 ==
  In1 : Inport
  Add : Sum  Inputs=+-
  Clock2 : Clock
  Constant : Constant
  Divide : Product  Inputs=*/
  Memory : Memory
  Relational Operator : RelationalOperator  OutDataTypeStr=boolean  RndMeth=Simplest
  Switch : Switch  Criteria=u2 > Threshold
  Out1 : Outport
  wires:
  Memory/1 -> Switch/3, Add/2
  Switch/1 -> Memory/1
  Add/1 -> Relational Operator/1
  Relational Operator/1 -> Switch/2, Out1/1
  Clock2/1 -> Add/1, Switch/1
  In1/1 -> Divide/2
  Constant/1 -> Divide/1
  Divide/1 -> Relational Operator/2

== system World_jessica_cs/BMW_X5_SUV_1/Frequency evaluator4 ==
  In1 : Inport
  Add : Sum  Inputs=+-
  Clock2 : Clock
  Constant : Constant
  Divide : Product  Inputs=*/
  Memory : Memory
  Relational Operator : RelationalOperator  OutDataTypeStr=boolean  RndMeth=Simplest
  Switch : Switch  Criteria=u2 > Threshold
  Out1 : Outport
  wires:
  Memory/1 -> Switch/3, Add/2
  Switch/1 -> Memory/1
  Add/1 -> Relational Operator/1
  Relational Operator/1 -> Switch/2, Out1/1
  Clock2/1 -> Add/1, Switch/1
  In1/1 -> Divide/2
  Constant/1 -> Divide/1
  Divide/1 -> Relational Operator/2

== system World_jessica_cs/BMW_X5_SUV_1/Frequency evaluator5 ==
  In1 : Inport
  Add : Sum  Inputs=+-
  Clock2 : Clock
  Constant : Constant
  Divide : Product  Inputs=*/
  Memory : Memory
  Relational Operator : RelationalOperator  OutDataTypeStr=boolean  RndMeth=Simplest
  Switch : Switch  Criteria=u2 > Threshold
  Out1 : Outport
  wires:
  Memory/1 -> Switch/3, Add/2
  Switch/1 -> Memory/1
  Add/1 -> Relational Operator/1
  Relational Operator/1 -> Switch/2, Out1/1
  Clock2/1 -> Add/1, Switch/1
  In1/1 -> Divide/2
  Constant/1 -> Divide/1
  Divide/1 -> Relational Operator/2

== system World_jessica_cs/BMW_X5_SUV_1/Frequency evaluator6 ==
  In1 : Inport
  Add : Sum  Inputs=+-
  Clock2 : Clock
  Constant : Constant
  Divide : Product  Inputs=*/
  Memory : Memory
  Relational Operator : RelationalOperator  OutDataTypeStr=boolean  RndMeth=Simplest
  Switch : Switch  Criteria=u2 > Threshold
  Out1 : Outport
  wires:
  Divide/1 -> Relational Operator/2
  Constant/1 -> Divide/1
  In1/1 -> Divide/2
  Clock2/1 -> Switch/1, Add/1
  Relational Operator/1 -> Out1/1, Switch/2
  Add/1 -> Relational Operator/1
  Switch/1 -> Memory/1
  Memory/1 -> Add/2, Switch/3

== system World_jessica_cs/BMW_X5_SUV_1/Frequency evaluator7 ==
  In1 : Inport
  Add : Sum  Inputs=+-
  Clock2 : Clock
  Constant : Constant
  Divide : Product  Inputs=*/
  Memory : Memory
  Relational Operator : RelationalOperator  OutDataTypeStr=boolean  RndMeth=Simplest
  Switch : Switch  Criteria=u2 > Threshold
  Out1 : Outport
  wires:
  Divide/1 -> Relational Operator/2
  Constant/1 -> Divide/1
  In1/1 -> Divide/2
  Clock2/1 -> Switch/1, Add/1
  Relational Operator/1 -> Out1/1, Switch/2
  Add/1 -> Relational Operator/1
  Switch/1 -> Memory/1
  Memory/1 -> Add/2, Switch/3

== system World_jessica_cs/BMW_X5_SUV_1/HumViewCamera_CM_Demux ==
  In1 : Inport
  Selector : Selector  NumberOfDimensions=2  InputPortWidth=3  IndexOptions=Index vector (dialog),Index vector (dialog)  Indices=-1,1:hres  OutputSizes=1,1
  Selector1 : Selector  NumberOfDimensions=2  InputPortWidth=3  IndexOptions=Index vector (dialog),Index vector (dialog)  Indices=-1,hres+1:hres*2  OutputSizes=1,1
  Selector2 : Selector  NumberOfDimensions=2  InputPortWidth=3  IndexOptions=Index vector (dialog),Index vector (dialog)  Indices=-1,hres*2+1:hres*3  OutputSizes=1,1
  R : Outport
  G : Outport  Port=2
  B : Outport  Port=3
  wires:
  In1/1 -> Selector1/1, Selector/1, Selector2/1
  Selector/1 -> R/1
  Selector1/1 -> G/1
  Selector2/1 -> B/1

== system World_jessica_cs/BMW_X5_SUV_1/PointCloudSensor_1_Angles_Demux ==
  In2 : Inport
  Selector : Selector  NumberOfDimensions=2  InputPortWidth=3  IndexOptions=Index vector (dialog),Index vector (dialog)  Indices=-1,offset+1:(offset+hres)  OutputSizes=1,1
  Selector1 : Selector  NumberOfDimensions=2  InputPortWidth=3  IndexOptions=Index vector (dialog),Index vector (dialog)  Indices=-1,(offset+hres+1):(offset+2*hres)  OutputSizes=1,1
  Theta : Outport
  Phi : Outport  Port=2
  wires:
  Selector1/1 -> Phi/1
  Selector/1 -> Theta/1
  In2/1 -> Selector/1, Selector1/1

== system World_jessica_cs/BMW_X5_SUV_1/PointCloudSensor_1_Intensity_Demux ==
  In1 : Inport
  Selector3 : Selector  NumberOfDimensions=2  InputPortWidth=3  IndexOptions=Index vector (dialog),Index vector (dialog)  Indices=-1,offset+1:(offset+hres)  OutputSizes=1,1
  Intensity : Outport
  wires:
  Selector3/1 -> Intensity/1
  In1/1 -> Selector3/1

== system World_jessica_cs/BMW_X5_SUV_1/PointCloudSensor_1_Range_Demux ==
  In1 : Inport
  Selector : Selector  NumberOfDimensions=2  InputPortWidth=3  IndexOptions=Index vector (dialog),Index vector (dialog)  Indices=-1,offset+1:(offset+hres)  OutputSizes=1,1
  Range : Outport
  wires:
  Selector/1 -> Range/1
  In1/1 -> Selector/1

== system World_jessica_cs/BMW_X5_SUV_1/PointCloudSensor_2_Angles_Demux ==
  In2 : Inport
  Selector : Selector  NumberOfDimensions=2  InputPortWidth=3  IndexOptions=Index vector (dialog),Index vector (dialog)  Indices=-1,offset+1:(offset+hres)  OutputSizes=1,1
  Selector1 : Selector  NumberOfDimensions=2  InputPortWidth=3  IndexOptions=Index vector (dialog),Index vector (dialog)  Indices=-1,(offset+hres+1):(offset+2*hres)  OutputSizes=1,1
  Theta : Outport
  Phi : Outport  Port=2
  wires:
  Selector1/1 -> Phi/1
  Selector/1 -> Theta/1
  In2/1 -> Selector/1, Selector1/1

== system World_jessica_cs/BMW_X5_SUV_1/PointCloudSensor_2_Intensity_Demux ==
  In1 : Inport
  Selector3 : Selector  NumberOfDimensions=2  InputPortWidth=3  IndexOptions=Index vector (dialog),Index vector (dialog)  Indices=-1,offset+1:(offset+hres)  OutputSizes=1,1
  Intensity : Outport
  wires:
  Selector3/1 -> Intensity/1
  In1/1 -> Selector3/1

== system World_jessica_cs/BMW_X5_SUV_1/PointCloudSensor_2_Range_Demux ==
  In1 : Inport
  Selector : Selector  NumberOfDimensions=2  InputPortWidth=3  IndexOptions=Index vector (dialog),Index vector (dialog)  Indices=-1,offset+1:(offset+hres)  OutputSizes=1,1
  Range : Outport
  wires:
  Selector/1 -> Range/1
  In1/1 -> Selector/1

== system World_jessica_cs/BMW_X5_SUV_1/PointCloudSensor_3_Angles_Demux ==
  In2 : Inport
  Selector : Selector  NumberOfDimensions=2  InputPortWidth=3  IndexOptions=Index vector (dialog),Index vector (dialog)  Indices=-1,offset+1:(offset+hres)  OutputSizes=1,1
  Selector1 : Selector  NumberOfDimensions=2  InputPortWidth=3  IndexOptions=Index vector (dialog),Index vector (dialog)  Indices=-1,(offset+hres+1):(offset+2*hres)  OutputSizes=1,1
  Theta : Outport
  Phi : Outport  Port=2
  wires:
  Selector1/1 -> Phi/1
  Selector/1 -> Theta/1
  In2/1 -> Selector/1, Selector1/1

== system World_jessica_cs/BMW_X5_SUV_1/PointCloudSensor_3_Intensity_Demux ==
  In1 : Inport
  Selector3 : Selector  NumberOfDimensions=2  InputPortWidth=3  IndexOptions=Index vector (dialog),Index vector (dialog)  Indices=-1,offset+1:(offset+hres)  OutputSizes=1,1
  Intensity : Outport
  wires:
  Selector3/1 -> Intensity/1
  In1/1 -> Selector3/1

== system World_jessica_cs/BMW_X5_SUV_1/PointCloudSensor_3_Range_Demux ==
  In1 : Inport
  Selector : Selector  NumberOfDimensions=2  InputPortWidth=3  IndexOptions=Index vector (dialog),Index vector (dialog)  Indices=-1,offset+1:(offset+hres)  OutputSizes=1,1
  Range : Outport
  wires:
  Selector/1 -> Range/1
  In1/1 -> Selector/1

== system World_jessica_cs/BMW_X5_SUV_1/PointCloudSensor_4_Angles_Demux ==
  In2 : Inport
  Selector : Selector  NumberOfDimensions=2  InputPortWidth=3  IndexOptions=Index vector (dialog),Index vector (dialog)  Indices=-1,offset+1:(offset+hres)  OutputSizes=1,1
  Selector1 : Selector  NumberOfDimensions=2  InputPortWidth=3  IndexOptions=Index vector (dialog),Index vector (dialog)  Indices=-1,(offset+hres+1):(offset+2*hres)  OutputSizes=1,1
  Theta : Outport
  Phi : Outport  Port=2
  wires:
  Selector1/1 -> Phi/1
  Selector/1 -> Theta/1
  In2/1 -> Selector/1, Selector1/1

== system World_jessica_cs/BMW_X5_SUV_1/PointCloudSensor_4_Intensity_Demux ==
  In1 : Inport
  Selector3 : Selector  NumberOfDimensions=2  InputPortWidth=3  IndexOptions=Index vector (dialog),Index vector (dialog)  Indices=-1,offset+1:(offset+hres)  OutputSizes=1,1
  Intensity : Outport
  wires:
  Selector3/1 -> Intensity/1
  In1/1 -> Selector3/1

== system World_jessica_cs/BMW_X5_SUV_1/PointCloudSensor_4_Range_Demux ==
  In1 : Inport
  Selector : Selector  NumberOfDimensions=2  InputPortWidth=3  IndexOptions=Index vector (dialog),Index vector (dialog)  Indices=-1,offset+1:(offset+hres)  OutputSizes=1,1
  Range : Outport
  wires:
  Selector/1 -> Range/1
  In1/1 -> Selector/1

== system World_jessica_cs/BMW_X5_SUV_1/Radar_1_Demux ==
  Radar : Inport
  Bus Selector1 : BusSelector  OutputSignals=ActiveBeamID[-],Range[m],DopplerVelocity[ms-1],DopplerVelocityX[ms-1],DopplerVelocityY[ms-1],DopplerVelocityZ[ms-1],Theta[deg],Phi[deg],TargetID[-],TargetTypeID[-],EnergyLoss[dB],Alpha[deg],Beta[deg]  OutputAsBus=on
  ScannerSensorLegacyBusConversion : PreScanUsefulBlocks/ScannerSensorLegacyBusConversion  MAXMESSAGES=MAXMESSAGES
  Radar Data : Outport
  wires:
  Bus Selector1/1 -> Radar Data/1
  ScannerSensorLegacyBusConversion/1 -> Bus Selector1/1
  Radar/1 -> ScannerSensorLegacyBusConversion/1

== system World_jessica_cs/BMW_X5_SUV_1/SELF_Demux ==
  SELF : Inport  OutDataTypeStr=Bus: PRESCAN_SELFSENSORDATA
  Bus Selector : BusSelector  OutputSignals=PositionX,PositionY,PositionZ,OrientationRoll,OrientationPitch,OrientationYaw,Velocity,Yaw_rate,Lat,Long,Alt
  Demux2 : Demux  Outputs=3
  Gain : Gain  Gain=180/pi
  Gain1 : Gain  Gain=180/pi
  Vector Concatenate1 : Concatenate  NumInputs=3
  compas converter : Subsystem
  x [m] : Outport
  y [m] : Outport  Port=2
  z [m] : Outport  Port=3
  rotx [deg] : Outport  Port=4
  roty [deg] : Outport  Port=5
  rotz [deg] : Outport  Port=6
  GPS lat [deg] : Outport  Port=7
  GPS long [deg] : Outport  Port=8
  GPS alt [m] : Outport  Port=9
  velocity [m/s] : Outport  Port=10
  heading [deg] : Outport  Port=11
  yaw rate [deg/s] : Outport  Port=12
  wires:
  Bus Selector/11 -> GPS alt [m]/1  "<Alt>"
  Bus Selector/10 -> GPS long [deg]/1  "<Long>"
  Bus Selector/9 -> GPS lat [deg]/1  "<Lat>"
  Bus Selector/8 -> Gain1/1  "<Yaw_rate>"
  Bus Selector/7 -> velocity [m/s]/1  "<Velocity>"
  Bus Selector/6 -> compas converter/1(rotz [rad]), Vector Concatenate1/3  "<OrientationYaw>"
  Bus Selector/5 -> Vector Concatenate1/2  "<OrientationPitch>"
  Bus Selector/4 -> Vector Concatenate1/1  "<OrientationRoll>"
  Vector Concatenate1/1 -> Gain/1
  Bus Selector/3 -> z [m]/1  "<PositionZ>"
  Bus Selector/2 -> y [m]/1  "<PositionY>"
  Bus Selector/1 -> x [m]/1  "<PositionX>"
  SELF/1 -> Bus Selector/1
  Gain/1 -> Demux2/1
  Demux2/1 -> rotx [deg]/1
  Demux2/2 -> roty [deg]/1
  Demux2/3 -> rotz [deg]/1
  compas converter/1(heading [deg]) -> heading [deg]/1
  Gain1/1 -> yaw rate [deg/s]/1

== system World_jessica_cs/Boy_150_1/Animation ==
  In1 : Inport
  Bus Creator : BusCreator  Inputs=2  OutDataTypeStr=Bus: PRESCAN_ANIMACTUATORDATA  NonVirtualBus=on
  Bus Selector : BusSelector  OutputSignals=VelocityX,VelocityY,VelocityZ
  Mux : Mux  Inputs=3
  animation mode : Subsystem
  elapsed track : Subsystem
  Out1 : Outport
  wires:
  animation mode/1(mode) -> Bus Creator/1  "Index"
  Bus Creator/1 -> Out1/1
  In1/1 -> Bus Selector/1
  elapsed track/1(s) -> Bus Creator/2  "Time"
  Bus Selector/3 -> Mux/3  "<VelocityZ>"
  Bus Selector/2 -> Mux/2  "<VelocityY>"
  Bus Selector/1 -> Mux/1  "<VelocityX>"
  Mux/1 -> animation mode/1(vel), elapsed track/1(vel)

== system World_jessica_cs/Boy_150_1/SELF_Demux ==
  SELF : Inport  OutDataTypeStr=Bus: PRESCAN_SELFSENSORDATA
  Bus Selector : BusSelector  OutputSignals=PositionX,PositionY,PositionZ,OrientationRoll,OrientationPitch,OrientationYaw,Velocity,Yaw_rate,Lat,Long,Alt
  Demux2 : Demux  Outputs=3
  Gain : Gain  Gain=180/pi
  Gain1 : Gain  Gain=180/pi
  Vector Concatenate1 : Concatenate  NumInputs=3
  compas converter : Subsystem
  x [m] : Outport
  y [m] : Outport  Port=2
  z [m] : Outport  Port=3
  rotx [deg] : Outport  Port=4
  roty [deg] : Outport  Port=5
  rotz [deg] : Outport  Port=6
  GPS lat [deg] : Outport  Port=7
  GPS long [deg] : Outport  Port=8
  GPS alt [m] : Outport  Port=9
  velocity [m/s] : Outport  Port=10
  heading [deg] : Outport  Port=11
  yaw rate [deg/s] : Outport  Port=12
  wires:
  Bus Selector/11 -> GPS alt [m]/1  "<Alt>"
  Bus Selector/10 -> GPS long [deg]/1  "<Long>"
  Bus Selector/9 -> GPS lat [deg]/1  "<Lat>"
  Bus Selector/8 -> Gain1/1  "<Yaw_rate>"
  Bus Selector/7 -> velocity [m/s]/1  "<Velocity>"
  Bus Selector/6 -> compas converter/1(rotz [rad]), Vector Concatenate1/3  "<OrientationYaw>"
  Bus Selector/5 -> Vector Concatenate1/2  "<OrientationPitch>"
  Bus Selector/4 -> Vector Concatenate1/1  "<OrientationRoll>"
  Vector Concatenate1/1 -> Gain/1
  Bus Selector/3 -> z [m]/1  "<PositionZ>"
  Bus Selector/2 -> y [m]/1  "<PositionY>"
  Bus Selector/1 -> x [m]/1  "<PositionX>"
  SELF/1 -> Bus Selector/1
  Gain/1 -> Demux2/1
  Demux2/1 -> rotx [deg]/1
  Demux2/2 -> roty [deg]/1
  Demux2/3 -> rotz [deg]/1
  compas converter/1(heading [deg]) -> heading [deg]/1
  Gain1/1 -> yaw rate [deg/s]/1

== system World_jessica_cs/Boy_150_1/VISUColorRegion_Lower_Body_Mux ==
  RGB [-,-,-] : Inport
  Bus Creator : BusCreator  Inputs=4  OutDataTypeStr=Bus: PRESCAN_COLOR_DATA  NonVirtualBus=on
  Constant : Constant  Value=255  OutDataTypeStr=uint8
  Data Type Conversion : DataTypeConversion  OutDataTypeStr=uint8
  Data Type Conversion1 : DataTypeConversion  OutDataTypeStr=uint8
  Data Type Conversion2 : DataTypeConversion  OutDataTypeStr=uint8
  Demux : Demux  Outputs=3
  ColorRegion : Outport  OutDataTypeStr=Bus: PRESCAN_COLOR_DATA  PortDimensions=1
  wires:
  Constant/1 -> Bus Creator/4  "A"
  Data Type Conversion2/1 -> Bus Creator/3  "B"
  Data Type Conversion1/1 -> Bus Creator/2  "G"
  Data Type Conversion/1 -> Bus Creator/1  "R"
  Demux/3 -> Data Type Conversion2/1  "B"
  Demux/2 -> Data Type Conversion1/1  "G"
  Demux/1 -> Data Type Conversion/1  "R"
  RGB [-,-,-]/1 -> Demux/1
  Bus Creator/1 -> ColorRegion/1
